simulink model "Basic_model_formulate"  (R2023b)
settings: Solver=VariableStepAuto  StartTime=0.0  StopTime=200  RelTol=1e-3
values from neighbouring files (symbols this model uses):
  Ac_real_system = zeros(N_state_variable_real_system)    [Real_system_initialization.m]
  Bc_real_system = zeros(N_state_variable_real_system,4)    [Real_system_initialization.m]
  Cc_real_system = eye(N_state_variable_real_system)    [Real_system_initialization.m]
  Dc_real_system = zeros(N_state_variable_real_system,1+1+1+1)    [Real_system_initialization.m]
settings Model: Creator=Administrator  LastModifiedBy=a1212313123
settings SolverCC: AlgebraicLoopSolver=TrustRegion
settings DataIOCC: ReturnWorkspaceOutputs=off
settings DebuggingCC: UnconnectedInputMsg=warning  UnconnectedOutputMsg=warning  UnconnectedLineMsg=warning  ArithmeticOperatorsInVariantConditions=warning
settings ModelReferenceCC: EnableRefExpFcnMdlSchedulingChecks=on
settings SFSimCC: SimUseLocalCustomCode=off  CustomCodeUndefinedFunction=UseInterfaceOnly
settings RTWCC: RTWUseLocalCustomCode=off

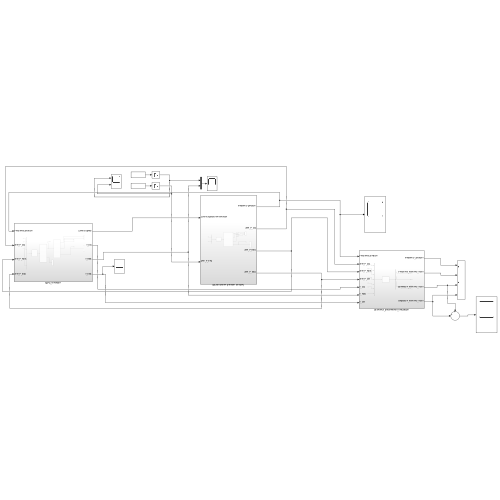
[thumbnail: Simulink's stored preview of the top-level diagram]
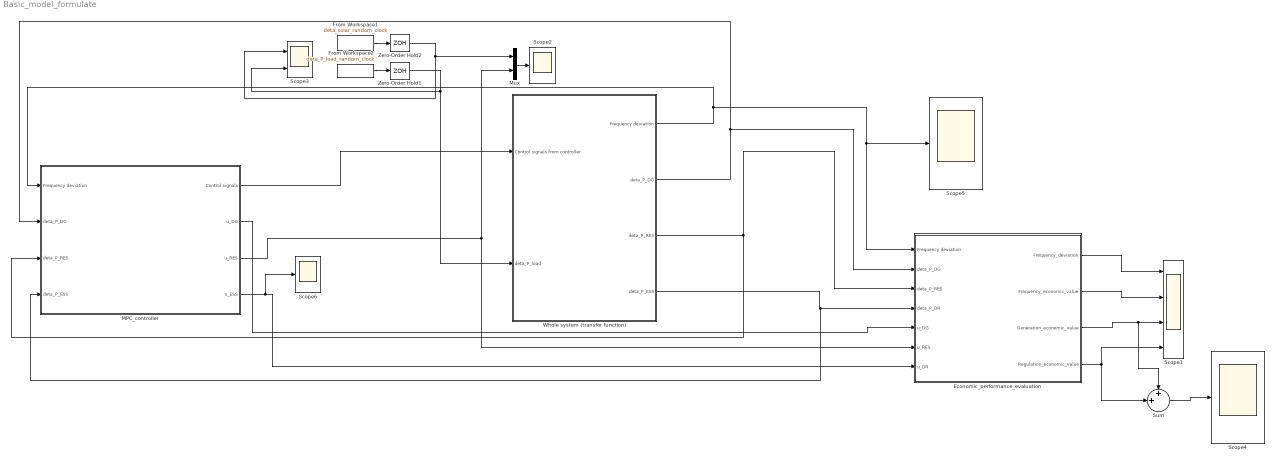
== system Basic_model_formulate ==
  Economic_performance_evaluation : Subsystem
  From Workspace1 : FromWorkspace  VariableName=deta_solar_random_clock
  From Workspace2 : FromWorkspace  VariableName=deta_P_load_random_clock
  MPC_controller : Subsystem
  Mux : Mux  Inputs=2
  Scope1 : Scope  NumInputPorts=4
  Scope{2,4..6} (4 alike) : Scope
  Scope3 : Scope  NumInputPorts=2
  Sum : Sum  Inputs=++|
  Whole system (transfer function) : Subsystem
  Zero-Order Hold1 : ZeroOrderHold  SampleTime=0.02
  Zero-Order Hold2 : ZeroOrderHold  SampleTime=0.02
  wires:
  From Workspace2/1 -> Zero-Order Hold1/1
  Zero-Order Hold1/1 -> Scope3/2, Whole system (transfer function)/2(deta_P_load)
  Whole system (transfer function)/1(Frequency deviation) -> MPC_controller/1(Frequency deviation), Economic_performance_evaluation/1(Frequency deviation), Scope5/1
  Whole system (transfer function)/2(deta_P_DG) -> MPC_controller/2(deta_P_DG), Economic_performance_evaluation/2(deta_P_DG)
  Whole system (transfer function)/3(deta_P_RES) -> Economic_performance_evaluation/3(deta_P_RES), MPC_controller/3(deta_P_RES)
  MPC_controller/1(Control signals) -> Whole system (transfer function)/1(Control signals from controller)
  From Workspace1/1 -> Zero-Order Hold2/1
  Zero-Order Hold2/1 -> Scope3/1, Mux/1
  MPC_controller/2(u_DG) -> Economic_performance_evaluation/5(u_DG)
  MPC_controller/3(u_RES) -> Economic_performance_evaluation/6(u_RES), Mux/2
  Whole system (transfer function)/4(deta_P_ESS) -> MPC_controller/4(deta_P_ESS), Economic_performance_evaluation/4(deta_P_DR)
  Economic_performance_evaluation/2(Frequency_economic_value) -> Scope1/2
  Economic_performance_evaluation/3(Generation_economic_value) -> Sum/1, Scope1/3
  Economic_performance_evaluation/1(Frequency_deviation) -> Scope1/1
  Sum/1 -> Scope4/1
  Mux/1 -> Scope2/1
  Economic_performance_evaluation/4(Regulation_economic_value) -> Sum/2, Scope1/4
  MPC_controller/4(u_ESS) -> Scope6/1, Economic_performance_evaluation/7(u_DR)

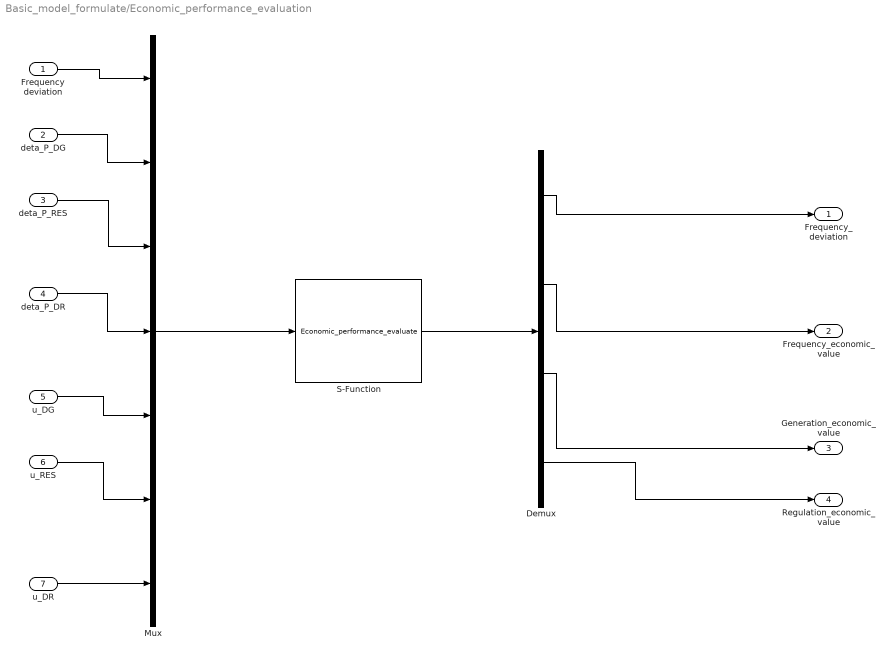
== system Basic_model_formulate/Economic_performance_evaluation ==
  Frequency deviation : Inport
  deta_P_DG : Inport  Port=2
  deta_P_RES : Inport  Port=3
  deta_P_DR : Inport  Port=4
  u_DG : Inport  Port=5
  u_RES : Inport  Port=6
  u_DR : Inport  Port=7
  Demux : Demux
  Mux : Mux  Inputs=7
  S-Function : S-Function  FunctionName=Economic_performance_evaluate  SFunctionDeploymentMode=off  EnableBusSupport=off
  Frequency_deviation : Outport  VectorParamsAs1DForOutWhenUnconnected=off
  Frequency_economic_value : Outport  Port=2  VectorParamsAs1DForOutWhenUnconnected=off
  Generation_economic_value : Outport  Port=3  VectorParamsAs1DForOutWhenUnconnected=off
  Regulation_economic_value : Outport  Port=4  VectorParamsAs1DForOutWhenUnconnected=off
  wires:
  Demux/2 -> Frequency_economic_value/1
  Demux/3 -> Generation_economic_value/1
  Demux/1 -> Frequency_deviation/1
  Mux/1 -> S-Function/1
  S-Function/1 -> Demux/1
  Demux/4 -> Regulation_economic_value/1
  Frequency deviation/1 -> Mux/1
  deta_P_DG/1 -> Mux/2
  deta_P_RES/1 -> Mux/3
  deta_P_DR/1 -> Mux/4
  u_DG/1 -> Mux/5
  u_RES/1 -> Mux/6
  u_DR/1 -> Mux/7

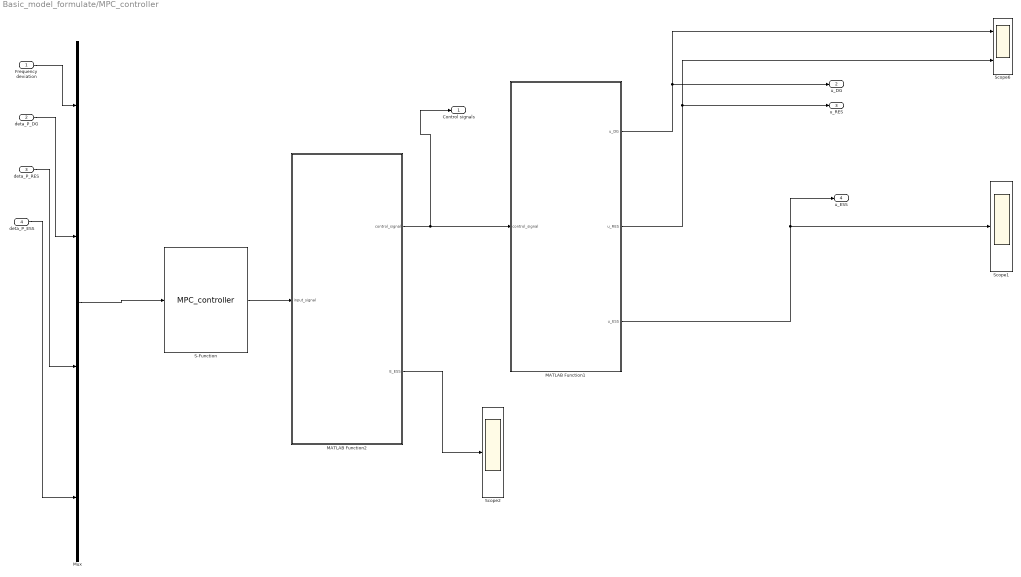
== system Basic_model_formulate/MPC_controller ==
  Frequency deviation : Inport
  deta_P_DG : Inport  Port=2
  deta_P_RES : Inport  Port=3
  deta_P_ESS : Inport  Port=4
  MATLAB Function1 : MATLAB Function  TreatAsAtomicUnit=on
  MATLAB Function2 : MATLAB Function  TreatAsAtomicUnit=on
  Mux : Mux
  S-Function : S-Function  FunctionName=MPC_controller  SFunctionDeploymentMode=off  EnableBusSupport=off
  Scope1 : Scope
  Scope2 : Scope
  Scope6 : Scope  NumInputPorts=2
  Control signals : Outport  VectorParamsAs1DForOutWhenUnconnected=off
  u_DG : Outport  Port=2  VectorParamsAs1DForOutWhenUnconnected=off
  u_RES : Outport  Port=3  VectorParamsAs1DForOutWhenUnconnected=off
  u_ESS : Outport  Port=4  VectorParamsAs1DForOutWhenUnconnected=off
  wires:
  deta_P_RES/1 -> Mux/3
  deta_P_ESS/1 -> Mux/4
  Mux/1 -> S-Function/1
  Frequency deviation/1 -> Mux/1
  deta_P_DG/1 -> Mux/2
  MATLAB Function1/1(u_DG) -> u_DG/1, Scope6/1
  MATLAB Function1/2(u_RES) -> u_RES/1, Scope6/2
  MATLAB Function1/3(u_ESS) -> u_ESS/1, Scope1/1
  S-Function/1 -> MATLAB Function2/1(input_signal)
  MATLAB Function2/1(control_signal) -> Control signals/1, MATLAB Function1/1(control_signal)
  MATLAB Function2/2(E_ESS) -> Scope2/1

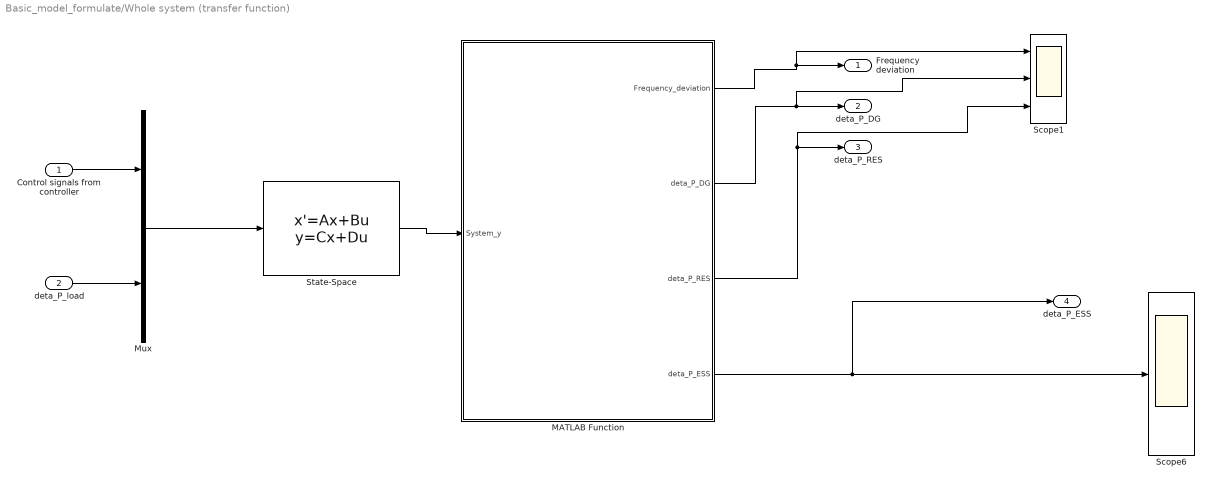
== system Basic_model_formulate/Whole system (transfer function) ==
  Control signals from controller : Inport
  deta_P_load : Inport  Port=2
  MATLAB Function : MATLAB Function  TreatAsAtomicUnit=on
  Mux : Mux  Inputs=2
  Scope1 : Scope  NumInputPorts=3
  Scope6 : Scope
  State-Space : StateSpace  A=Ac_real_system  B=Bc_real_system  C=Cc_real_system  D=Dc_real_system  InitialCondition=0
  Frequency deviation : Outport  VectorParamsAs1DForOutWhenUnconnected=off
  deta_P_DG : Outport  Port=2  VectorParamsAs1DForOutWhenUnconnected=off
  deta_P_RES : Outport  Port=3  VectorParamsAs1DForOutWhenUnconnected=off
  deta_P_ESS : Outport  Port=4  VectorParamsAs1DForOutWhenUnconnected=off
  wires:
  deta_P_load/1 -> Mux/2
  Control signals from controller/1 -> Mux/1
  Mux/1 -> State-Space/1
  State-Space/1 -> MATLAB Function/1(System_y)
  MATLAB Function/1(Frequency_deviation) -> Scope1/1, Frequency deviation/1
  MATLAB Function/2(deta_P_DG) -> Scope1/2, deta_P_DG/1
  MATLAB Function/3(deta_P_RES) -> Scope1/3, deta_P_RES/1
  MATLAB Function/4(deta_P_ESS) -> deta_P_ESS/1, Scope6/1

== matlab function Basic_model_formulate/MPC_controller/MATLAB Function2 ==
  data: input_signal input; control_signal output; E_ESS output
function [control_signal,E_ESS] = Classify_control_signal(input_signal)
    control_signal = input_signal(1:3);
    E_ESS = input_signal(4);
end

== matlab function Basic_model_formulate/Whole system (transfer function)/MATLAB Function ==
  data: System_y input; Frequency_deviation output; deta_P_DG output; deta_P_RES output; deta_P_ESS output
function [Frequency_deviation, deta_P_DG, deta_P_RES,deta_P_ESS] = Sampling_system_state(System_y)

Frequency_deviation=System_y(1);
deta_P_DG=System_y(2);
deta_P_RES=System_y(3);
deta_P_ESS = System_y(4); % 包含44个元素
end

== matlab function Basic_model_formulate/MPC_controller/MATLAB Function1 ==
  data: control_signal input; u_DG output; u_RES output; u_ESS output
function [u_DG,u_RES,u_ESS] = Classify_control_signal(control_signal)

    u_DG = control_signal(1);
    u_RES = control_signal(2);
    u_ESS = control_signal(3);
end
